simulink model "thyristor_firing"  (R2023b)
settings: Solver=VariableStepAuto  StartTime=0.0  StopTime=0.40  MaxStep=tstepMax  RelTol=1e-3
values from neighbouring files (symbols this model uses):
  alpha = (103*pi/180)*20e-3/(2*pi)    (= 0.00572222222222)    [thyristor.m]
  v_in = 15*sqrt(2)    [Q3_2.m]    (also in thyristor.m = 20)
undefined symbols (not defined in the file or in its folder): Ion, Lithium
libraries: spsThyristorLib x6, spsVoltageMeasurementLib x4, spsACVoltageSourceLib x3, spsBatteryLib x1, spsCurrentMeasurementLib x1, spsSeriesRLCBranchLib x1, sps_lib x1
settings Model: Creator=Emir  LastModifiedBy=abdulkadir

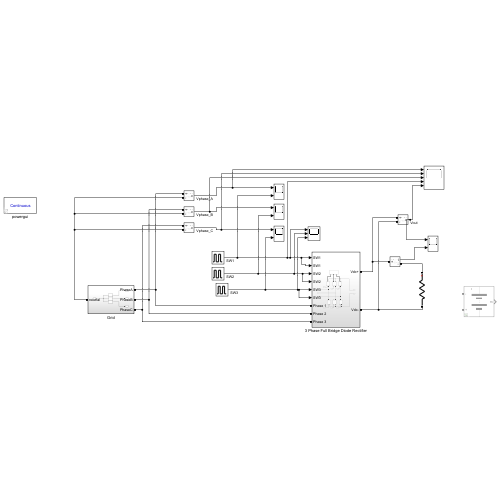
[thumbnail: Simulink's stored preview of the top-level diagram]
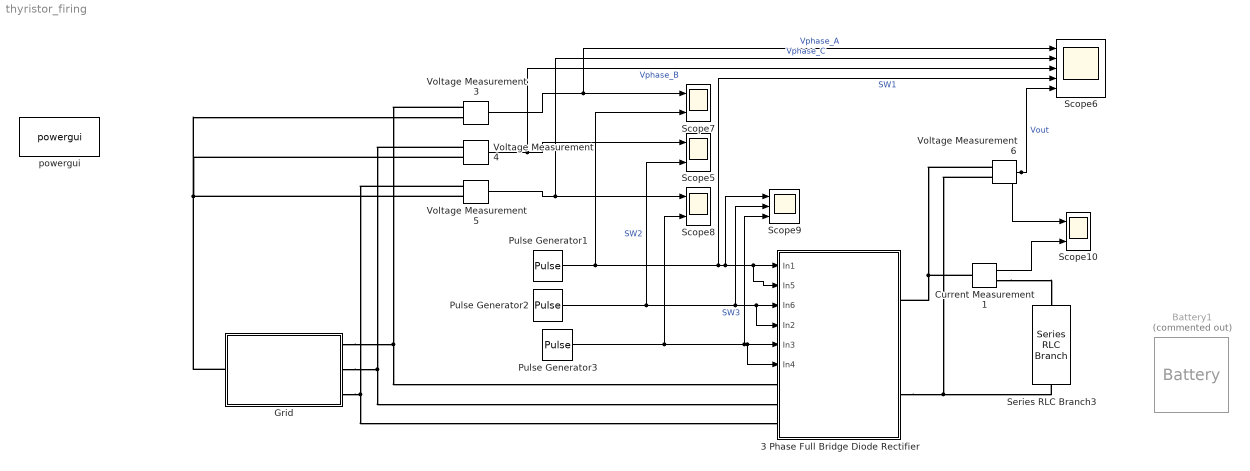
== system thyristor_firing ==
  3 Phase Full Bridge Diode Rectifier : Subsystem
  Battery1 : spsBatteryLib/Battery  Commented=on  BatType=Lithium-Ion  ShowTempParam=off  ThermalPreset=no  ShowAgeParam=off  NomV=7.2  NomQ=5.4  SOC=100  Batt_Tr=30  PresetModel=on  MaxQ=5.4  MinV=5.4  FullV=8.3807  Dis_rate=2.3478  R=0.013333  Normal_OP=4.8835  expZone="[7.7788      0.2653]"  current=[6.5 13 32.5]  Units=Time  Tci=20  NomT=20  T2=-30  MaxQ2=4.8  FullV2=7.1  Normal_OP2=5.655  expZone2="[6.58           1]"  Rca=0.6  ti=2000  Dp=0  Neq0=0  Tsim=1e6  Ta1=25  Qeol=5.4*0.9  Reol=0.013333*1.2  Char_age=[2.3478, 3]  Dis_age=[2.3478, 10]  N1=1500  N2=10500  N3=1000  N4=1400  Ta2=45  N5=950
  Current Measurement1 : spsCurrentMeasurementLib/Current Measurement  PhasorSimulation=off  OutputType=Complex  PSBequivalent=0
  Grid : Subsystem
  Pulse Generator1 : DiscretePulseGenerator  PulseType=Time based  Period=20e-3  PulseWidth=50  PhaseDelay=-20e-3/12 + alpha
  Pulse Generator2 : DiscretePulseGenerator  PulseType=Time based  Period=20e-3  PulseWidth=50  PhaseDelay=-20e-3/3+20e-3/12 + alpha
  Pulse Generator3 : DiscretePulseGenerator  PulseType=Time based  Period=20e-3  PulseWidth=50  PhaseDelay=-40e-3/3+20e-3/12 + alpha
  Scope{5,7..8,10} (4 alike) : Scope  NumInputPorts=2
  Scope6 : Scope  NumInputPorts=5
  Scope9 : Scope  NumInputPorts=3
  Series RLC Branch3 : spsSeriesRLCBranchLib/Series RLC Branch  LConnTagsString=__new0  RConnTagsString=__new0  BranchType=R  Resistance=1  Inductance=1e-3  SetiL0=off  InitialCurrent=0  Capacitance=1e-6  Setx0=off  InitialVoltage=0  Measurements=None
  Voltage Measurement{3..6} (4 alike) : spsVoltageMeasurementLib/Voltage Measurement  PhasorSimulation=off  OutputType=Complex  PSBequivalent=0
  powergui : sps_lib/powergui  Priority=1  SimulationMode=Continuous  SampleTime=50e-6  frequency=60  Iterations=50  frequencyindice=50  Pbase=100e6  ErrMax=1e-4  UnitsV=kV  UnitsW=MW  buscounter=0  FunctionMessages=off  echomessages=off  EnableUseOfTLC=off  CurrentSourceSwitches=off  DisableSnubberDevices=off  DisableRonSwitches=off  DisableVfSwitches=off  DisplayEquations=off  AutomaticDiscreteSolvers=off  SolverType=Tustin/Backward Euler (TBE)  Interpol=off  ExternalGateDelay=off  methode=off  Ts=100  x0status=blocks  SPID=on  SwTol=0  HookPort=off  NonlinearTolerance=1e-4  nMaxIteration=100  ContinueOnMaxIteration=off  RestoreLinks=warning  ResistiveCurrentMeasurement=off  Frange=[0:2:500]  Ylog=off  Xlog=on  ShowGrid=off  save=off  variable=ZData  structure=0  ZoomFFT=off  StartTime=0.0  cycles=1  DisplayStyle=1  fundamental=60  FreqAxis=off  MaxFrequency=1000  frequencyindicesteady=1  RmsSteady=1  display=off
  wires:
  Voltage Measurement4/1 -> Scope6/3, Scope5/1  "Vphase_B"
  Voltage Measurement5/1 -> Scope6/2, Scope8/1  "Vphase_C"
  Voltage Measurement3/1 -> Scope6/1, Scope7/1  "Vphase_A"
  Pulse Generator3/1 -> 3 Phase Full Bridge Diode Rectifier/5(In3), 3 Phase Full Bridge Diode Rectifier/6(In4), Scope9/3, Scope8/2  "SW3"
  Pulse Generator1/1 -> Scope7/2, Scope6/4, 3 Phase Full Bridge Diode Rectifier/2(In5), 3 Phase Full Bridge Diode Rectifier/1(In1), Scope9/1  "SW1"
  Pulse Generator2/1 -> Scope5/2, 3 Phase Full Bridge Diode Rectifier/3(In6), 3 Phase Full Bridge Diode Rectifier/4(In2), Scope9/2  "SW2"
  Current Measurement1/1 -> Scope10/2
  Voltage Measurement6/1 -> Scope10/1, Scope6/5  "Vout"
  connections:
  Grid/RConn1 -- Voltage Measurement3/LConn1 -- 3 Phase Full Bridge Diode Rectifier/LConn1
  Grid/RConn2 -- Voltage Measurement4/LConn1 -- 3 Phase Full Bridge Diode Rectifier/LConn2
  Grid/RConn3 -- Voltage Measurement5/LConn1 -- 3 Phase Full Bridge Diode Rectifier/LConn3
  Grid/LConn1 -- Voltage Measurement4/LConn2 -- Voltage Measurement3/LConn2 -- Voltage Measurement5/LConn2
  Voltage Measurement6/LConn1 -- Current Measurement1/LConn1 -- 3 Phase Full Bridge Diode Rectifier/RConn1
  3 Phase Full Bridge Diode Rectifier/RConn2 -- Voltage Measurement6/LConn2 -- Series RLC Branch3/RConn1
  Current Measurement1/RConn1 -- Series RLC Branch3/LConn1

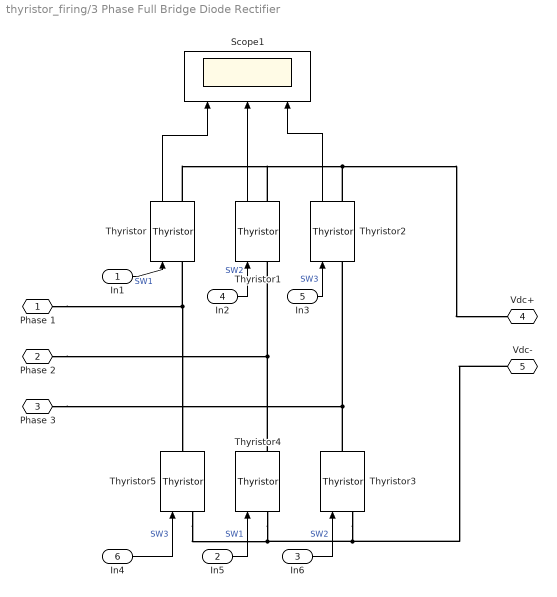
== system thyristor_firing/3 Phase Full Bridge Diode Rectifier ==
  In1 : Inport
  In5 : Inport  Port=2
  In6 : Inport  Port=3
  In2 : Inport  Port=4
  In3 : Inport  Port=5
  In4 : Inport  Port=6
  Scope1 : Scope  NumInputPorts=3
  Thyristor{,1..2,4} (4 alike) : spsThyristorLib/Thyristor  Ron=0.001  Lon=0  Vf=0.8  IC=0  Rs=500  Cs=250e-9  Measurements=on
  Thyristor3 : spsThyristorLib/Thyristor  Ron=0.001  Lon=0  Vf=0.8  IC=0  Rs=500  Cs=250e-9  Measurements=off
  Thyristor5 : spsThyristorLib/Thyristor  Ron=0.001  Lon=0  Vf=0.8  IC=0  Rs=500  Cs=250e-9  Measurements=off
  Phase 1 : PMIOPort  Side=Left
  Phase 2 : PMIOPort  Port=2  Side=Left
  Phase 3 : PMIOPort  Port=3  Side=Left
  Vdc+ : PMIOPort  Port=4  Side=Right
  Vdc- : PMIOPort  Port=5  Side=Right
  wires:
  In1/1 -> Thyristor/1  "SW1"
  In2/1 -> Thyristor1/1  "SW2"
  In3/1 -> Thyristor2/1  "SW3"
  In4/1 -> Thyristor5/1  "SW3"
  In5/1 -> Thyristor4/1  "SW1"
  In6/1 -> Thyristor3/1  "SW2"
  Thyristor/1 -> Scope1/1
  Thyristor1/1 -> Scope1/2
  Thyristor2/1 -> Scope1/3
  connections:
  Phase 2/RConn1 -- Thyristor1/LConn1 -- Thyristor4/RConn1
  Phase 3/RConn1 -- Thyristor2/LConn1 -- Thyristor3/RConn1
  Phase 1/RConn1 -- Thyristor5/RConn1 -- Thyristor/LConn1
  Vdc-/RConn1 -- Thyristor3/LConn1 -- Thyristor5/LConn1 -- Thyristor4/LConn1
  Thyristor1/RConn1 -- Thyristor/RConn1 -- Thyristor2/RConn1 -- Vdc+/RConn1

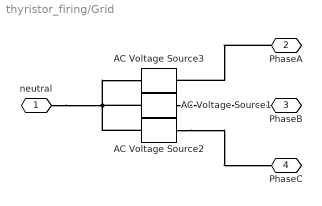
== system thyristor_firing/Grid ==
  AC Voltage Source1 : spsACVoltageSourceLib/AC Voltage Source  Amplitude=v_in  Phase=120  Frequency=50  SampleTime=0  Measurements=None  BusType=swing  Pref=10e3  Qref=0  Qmin=-inf  Qmax=+inf
  AC Voltage Source2 : spsACVoltageSourceLib/AC Voltage Source  Amplitude=v_in  Phase=240  Frequency=50  SampleTime=0  Measurements=None  BusType=swing  Pref=10e3  Qref=0  Qmin=-inf  Qmax=+inf
  AC Voltage Source3 : spsACVoltageSourceLib/AC Voltage Source  Amplitude=v_in  Phase=0  Frequency=50  SampleTime=0  Measurements=None  BusType=swing  Pref=10e3  Qref=0  Qmin=-inf  Qmax=+inf
  neutral : PMIOPort  Side=Left
  PhaseA : PMIOPort  Port=2  Side=Right
  PhaseB : PMIOPort  Port=3  Side=Right
  PhaseC : PMIOPort  Port=4  Side=Right
  connections:
  AC Voltage Source1/RConn1 -- PhaseB/RConn1
  PhaseA/RConn1 -- AC Voltage Source3/RConn1
  AC Voltage Source2/RConn1 -- PhaseC/RConn1
  neutral/RConn1 -- AC Voltage Source3/LConn1 -- AC Voltage Source2/LConn1 -- AC Voltage Source1/LConn1
